simulink model "Control_planta_no_lineal_y_NN_mejor"  (R2023b)
settings: Solver=ode45  StartTime=0.0  StopTime=5000  RelTol=1e-3
values from neighbouring files (symbols this model uses):
  D = 0    [control_pid_tuning.m]
libraries: neural x98, simulink x9
(part 4 of 5)

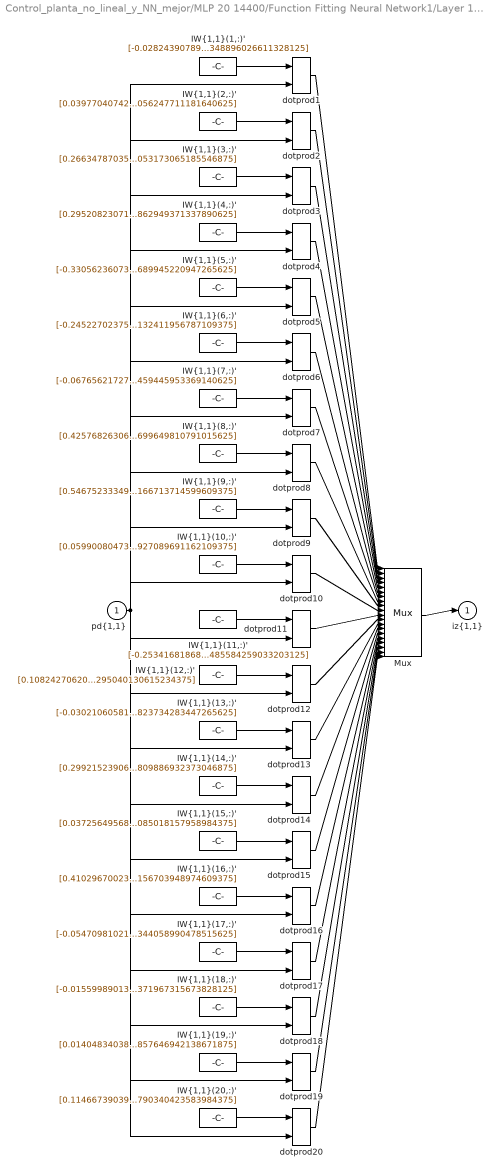
== system Control_planta_no_lineal_y_NN_mejor/MLP 20 14400/Function Fitting Neural Network1/Layer 1/IW{1,1} ==
  "pd{1,1}" : Inport  PortDimensions=11
      mask Display: e = 0.06;c1 = [120 230 180]/255;c2 = ([120 230 180]+0)/(256+128);c3 = ([120 230 180]+128)/(256+128);patch([0 1 1 0],[0 0 1 1],c1);patch([0 1 1 1-e 1-e 0+e],[0 0 1 1-e 0+e 0+e],c2);patch([0 0 1 1-e 0+e 0+e],[0 1 1 1-e 1-e 0+e],c3);plot([0 1 1 0 0],[0 0 1 1 0]);
  "IW{1,1}(1,:)'" : Constant  Value=[-0.028243907895395957419193422310854657553136348724365234375;0.005191973974844788126958849971970266778953373432159423828125;0.13337941289357180263408508835709653794765472412109375;0.069147078104058790071206885841093026101589202880859375;0.09470631313108242299581007728193071670830249786376953125;-0.0034271328340436456143247578864929892006330192089080810546875;0.04562563126758666098847783132441691122949123382568359375;-0.1381497395252362092588072073340299539268016815185546875;0.06431424914707263573721007787753478623926639556884765625;0.025641370199923095574146003627902246080338954925537109375;0.055434669391018993878095244554060627706348896026611328125]
      mask Display: e = 0.06;c1 = [120 150 230]/255;c2 = ([120 150 230]+0)/383;c3 = ([120 150 230]+128)/383;patch([0 1 1 0],[0 0 1 1],c1);patch([0 1 1 1-e 1-e 0+e],[0 0 1 1-e 0+e 0+e],c2);patch([0 0 1 1-e 0+e 0+e],[0 1 1 1-e 1-e 0+e],c3);plot([0 1 1 0 0],[0 0 1 1 0]);disp('Weights');
  "IW{1,1}(10,:)'" : Constant  Value=[0.059900804730095118244559415643379907123744487762451171875;0.0197715008122807678336840808697161264717578887939453125;0.04772829613961322714477120143783395178616046905517578125;-0.0932621366212354196978395748374168761074542999267578125;0.11487215483931519088844908083046902902424335479736328125;-0.0811079282463227635435742968184058554470539093017578125;-0.041933844459557438610897150965683977119624614715576171875;0.1459137174109600143534493099650717340409755706787109375;-0.0001450925426568216449439707727009363225079141557216644287109375;-0.007609474599997727468914110460218580556102097034454345703125;0.08578395140804272178680633942349231801927089691162109375]
      mask Display: e = 0.06;c1 = [120 150 230]/255;c2 = ([120 150 230]+0)/383;c3 = ([120 150 230]+128)/383;patch([0 1 1 0],[0 0 1 1],c1);patch([0 1 1 1-e 1-e 0+e],[0 0 1 1-e 0+e 0+e],c2);patch([0 0 1 1-e 0+e 0+e],[0 1 1 1-e 1-e 0+e],c3);plot([0 1 1 0 0],[0 0 1 1 0]);disp('Weights');
  "IW{1,1}(11,:)'" : Constant  Value=[-0.253416818681620303888024636762565933167934417724609375;0.052896434451703618073725721160371904261410236358642578125;0.068915348393704001228599054229562170803546905517578125;-0.09788049413072692772619376455622841604053974151611328125;0.057178838120491182195337387383915483951568603515625;0.10728410449795654224569574353154166601598262786865234375;0.0203502020408309301779947730892672552727162837982177734375;0.00125229069658645592207080188273948806454427540302276611328125;-0.14408483033475272261370037085725925862789154052734375;0.046135919620093245041569929298930219374597072601318359375;0.048354326720816971640903858542515081353485584259033203125]
      mask Display: e = 0.06;c1 = [120 150 230]/255;c2 = ([120 150 230]+0)/383;c3 = ([120 150 230]+128)/383;patch([0 1 1 0],[0 0 1 1],c1);patch([0 1 1 1-e 1-e 0+e],[0 0 1 1-e 0+e 0+e],c2);patch([0 0 1 1-e 0+e 0+e],[0 1 1 1-e 1-e 0+e],c3);plot([0 1 1 0 0],[0 0 1 1 0]);disp('Weights');
  "IW{1,1}(12,:)'" : Constant  Value=[0.1082427062098151038238569299210212193429470062255859375;-0.10783347592795040903457248759877984412014484405517578125;0.04932416990094290465407311785384081304073333740234375;0.1176909494571356240566473161379690282046794891357421875;0.056625605240315700361630746328955865465104579925537109375;0.125540484944335284378524875137372873723506927490234375;-0.009781079733660345831847138242665096186101436614990234375;0.0033784039907568054646180844002856247243471443653106689453125;-0.0201388726176935060896422413634354597888886928558349609375;-0.13223024952066808612727299987454898655414581298828125;0.106353782749821712538818019311293028295040130615234375]
      mask Display: e = 0.06;c1 = [120 150 230]/255;c2 = ([120 150 230]+0)/383;c3 = ([120 150 230]+128)/383;patch([0 1 1 0],[0 0 1 1],c1);patch([0 1 1 1-e 1-e 0+e],[0 0 1 1-e 0+e 0+e],c2);patch([0 0 1 1-e 0+e 0+e],[0 1 1 1-e 1-e 0+e],c3);plot([0 1 1 0 0],[0 0 1 1 0]);disp('Weights');
  "IW{1,1}(13,:)'" : Constant  Value=[-0.0302106058159601724433240832468072767369449138641357421875;-0.01083473636973667809935140127208796911872923374176025390625;0.00872722778809984812975475421126247965730726718902587890625;0.1694700438931255048746749025667668320238590240478515625;-0.055846650548267817715242244958062656223773956298828125;0.0683259083119855115118213007008307613432407379150390625;0.09901740039771596280093746145212207920849323272705078125;-0.0034830733886535903721937135202324498095549643039703369140625;0.086367876376208629896069624010124243795871734619140625;-0.0785352645771759394488498173814150504767894744873046875;0.11200836262547832211655673972927615977823734283447265625]
      mask Display: e = 0.06;c1 = [120 150 230]/255;c2 = ([120 150 230]+0)/383;c3 = ([120 150 230]+128)/383;patch([0 1 1 0],[0 0 1 1],c1);patch([0 1 1 1-e 1-e 0+e],[0 0 1 1-e 0+e 0+e],c2);patch([0 0 1 1-e 0+e 0+e],[0 1 1 1-e 1-e 0+e],c3);plot([0 1 1 0 0],[0 0 1 1 0]);disp('Weights');
  "IW{1,1}(14,:)'" : Constant  Value=[0.299215239064117122236297063864185474812984466552734375;-0.227303056462553942917992344519007019698619842529296875;-0.0246028750168633993100630874550915905274450778961181640625;0.0274141703222423004093766252253772108815610408782958984375;-0.0728212599418223138769690194749273359775543212890625;0.128567286087202525823869336818461306393146514892578125;-0.06510115768746389808274699362300452776253223419189453125;-0.0227893282940125098401384917679024511016905307769775390625;-0.0116248315098215031226924764951036195270717144012451171875;0.10342143834431290205788656066943076439201831817626953125;-0.057548270876921485406096934411834808997809886932373046875]
      mask Display: e = 0.06;c1 = [120 150 230]/255;c2 = ([120 150 230]+0)/383;c3 = ([120 150 230]+128)/383;patch([0 1 1 0],[0 0 1 1],c1);patch([0 1 1 1-e 1-e 0+e],[0 0 1 1-e 0+e 0+e],c2);patch([0 0 1 1-e 0+e 0+e],[0 1 1 1-e 1-e 0+e],c3);plot([0 1 1 0 0],[0 0 1 1 0]);disp('Weights');
  "IW{1,1}(15,:)'" : Constant  Value=[0.03725649568679145762217785886605270206928253173828125;0.058076084950603797107948622624462586827576160430908203125;-0.1269729602577863991630380269270972348749637603759765625;-0.01786746093381354205664734990932629443705081939697265625;-0.1569183017659522005882166695300838910043239593505859375;0.03235562642280716272313867420962196774780750274658203125;0.06457104482191818040082154084302601404488086700439453125;0.006190341039861292464496766996262522297911345958709716796875;-0.06269301714694208715883405602653510868549346923828125;-0.0645635039482781170061542752591776661574840545654296875;-0.103030060916822152616845187367289327085018157958984375]
      mask Display: e = 0.06;c1 = [120 150 230]/255;c2 = ([120 150 230]+0)/383;c3 = ([120 150 230]+128)/383;patch([0 1 1 0],[0 0 1 1],c1);patch([0 1 1 1-e 1-e 0+e],[0 0 1 1-e 0+e 0+e],c2);patch([0 0 1 1-e 0+e 0+e],[0 1 1 1-e 1-e 0+e],c3);plot([0 1 1 0 0],[0 0 1 1 0]);disp('Weights');
  "IW{1,1}(16,:)'" : Constant  Value=[0.41029670023388609134684656964964233338832855224609375;-0.054189782981134991535210332358474261127412319183349609375;-0.070172139747485762217849014632520265877246856689453125;-0.00901359172674678042758156237823641276918351650238037109375;-0.0008664644738628286997628169530116792884655296802520751953125;-0.0839314079297433790483040638719103299081325531005859375;-0.0105366135053931476994737437280491576530039310455322265625;0.0669426632220568584852316007527406327426433563232421875;-0.0782121647827017929532900097910896874964237213134765625;0.01064688551336578740957872213357404689304530620574951171875;0.0767344182627665849505405049058026634156703948974609375]
      mask Display: e = 0.06;c1 = [120 150 230]/255;c2 = ([120 150 230]+0)/383;c3 = ([120 150 230]+128)/383;patch([0 1 1 0],[0 0 1 1],c1);patch([0 1 1 1-e 1-e 0+e],[0 0 1 1-e 0+e 0+e],c2);patch([0 0 1 1-e 0+e 0+e],[0 1 1 1-e 1-e 0+e],c3);plot([0 1 1 0 0],[0 0 1 1 0]);disp('Weights');
  "IW{1,1}(17,:)'" : Constant  Value=[-0.054709810218583732055463997312472201883792877197265625;-0.058222078569764669497832443312290706671774387359619140625;0.0272915548239388953966066964085257495753467082977294921875;-0.002060889782607545385462177733870703377760946750640869140625;0.045200565384666151202974759826247463934123516082763671875;0.036566709240253382484642230565441423095762729644775390625;0.048434724470805601281853114414843730628490447998046875;0.1485881234961840269281907467302517034113407135009765625;-0.08280095269822450310126527028842247091233730316162109375;-0.01401815776626045596808811666278415941633284091949462890625;-0.100518799537367531371501172543503344058990478515625]
      mask Display: e = 0.06;c1 = [120 150 230]/255;c2 = ([120 150 230]+0)/383;c3 = ([120 150 230]+128)/383;patch([0 1 1 0],[0 0 1 1],c1);patch([0 1 1 1-e 1-e 0+e],[0 0 1 1-e 0+e 0+e],c2);patch([0 0 1 1-e 0+e 0+e],[0 1 1 1-e 1-e 0+e],c3);plot([0 1 1 0 0],[0 0 1 1 0]);disp('Weights');
  "IW{1,1}(18,:)'" : Constant  Value=[-0.01559989013582755400244561627687289728783071041107177734375;0.1058168090239341996294797354494221508502960205078125;-0.06821074930672578473522804642925621010363101959228515625;0.06328489319008401281507758540101349353790283203125;0.054756660574826011844695727859289036132395267486572265625;-0.053094792779526507608967023088553105480968952178955078125;0.025051428903148105498122077960942988283932209014892578125;-0.0230630997120841833847304513938070158474147319793701171875;0.159954775259797787878568442465621046721935272216796875;0.1668385232983627675107385357478051446378231048583984375;-0.1532613816918442228853791675646789371967315673828125]
      mask Display: e = 0.06;c1 = [120 150 230]/255;c2 = ([120 150 230]+0)/383;c3 = ([120 150 230]+128)/383;patch([0 1 1 0],[0 0 1 1],c1);patch([0 1 1 1-e 1-e 0+e],[0 0 1 1-e 0+e 0+e],c2);patch([0 0 1 1-e 0+e 0+e],[0 1 1 1-e 1-e 0+e],c3);plot([0 1 1 0 0],[0 0 1 1 0]);disp('Weights');
  "IW{1,1}(19,:)'" : Constant  Value=[0.01404834038980782608130315480821082019247114658355712890625;0.11681275441382070467977172256723861210048198699951171875;-0.074121670900885894273102394436136819422245025634765625;0.06853045999625316520020845700855716131627559661865234375;-0.0675103126368933048606635338728665374219417572021484375;0.10978393057352721362551761785653070546686649322509765625;-0.0695348327221847750667649279421311803162097930908203125;-0.07792378774692478027308339960654848255217075347900390625;0.03166961717159981481994890373243833892047405242919921875;0.10311534148308466873888988857288495637476444244384765625;-0.07671983312766754437017624468353460542857646942138671875]
      mask Display: e = 0.06;c1 = [120 150 230]/255;c2 = ([120 150 230]+0)/383;c3 = ([120 150 230]+128)/383;patch([0 1 1 0],[0 0 1 1],c1);patch([0 1 1 1-e 1-e 0+e],[0 0 1 1-e 0+e 0+e],c2);patch([0 0 1 1-e 0+e 0+e],[0 1 1 1-e 1-e 0+e],c3);plot([0 1 1 0 0],[0 0 1 1 0]);disp('Weights');
  "IW{1,1}(2,:)'" : Constant  Value=[0.039770407428281522033142181271614390425384044647216796875;-0.0245520760030410005458900712937975185923278331756591796875;0.03863350951806406030630824943727930076420307159423828125;0.117783072418614576104545221824082545936107635498046875;-0.091235315425064966721180326203466393053531646728515625;0.07428623396314408544593987926418776623904705047607421875;-0.076683739339302114945695620917831547558307647705078125;0.0269126755066263871618570391319735790602862834930419921875;-0.1583206985996788163095772006272454746067523956298828125;-0.166224771381416724924662275952869094908237457275390625;-0.0061015994473339052461824394413270056247711181640625]
      mask Display: e = 0.06;c1 = [120 150 230]/255;c2 = ([120 150 230]+0)/383;c3 = ([120 150 230]+128)/383;patch([0 1 1 0],[0 0 1 1],c1);patch([0 1 1 1-e 1-e 0+e],[0 0 1 1-e 0+e 0+e],c2);patch([0 0 1 1-e 0+e 0+e],[0 1 1 1-e 1-e 0+e],c3);plot([0 1 1 0 0],[0 0 1 1 0]);disp('Weights');
  "IW{1,1}(20,:)'" : Constant  Value=[0.11466739039623814744306429247444611974060535430908203125;-0.09303822905549240240841157856266363523900508880615234375;-0.0109706113092430633526586092330035171471536159515380859375;0.121986783925877972922791059318115003407001495361328125;0.005601834845350785012374483784469703095965087413787841796875;0.08696978354123073573500590782714425586163997650146484375;-0.0828842101220638449721178631079965271055698394775390625;-0.0932241771186295142825883885961957275867462158203125;0.049048714470215575012002062749161268584430217742919921875;0.0778398446714923253342277575939078815281391143798828125;0.0807200930695547158588709635296254418790340423583984375]
      mask Display: e = 0.06;c1 = [120 150 230]/255;c2 = ([120 150 230]+0)/383;c3 = ([120 150 230]+128)/383;patch([0 1 1 0],[0 0 1 1],c1);patch([0 1 1 1-e 1-e 0+e],[0 0 1 1-e 0+e 0+e],c2);patch([0 0 1 1-e 0+e 0+e],[0 1 1 1-e 1-e 0+e],c3);plot([0 1 1 0 0],[0 0 1 1 0]);disp('Weights');
  "IW{1,1}(3,:)'" : Constant  Value=[0.266347870359112837146398078402853570878505706787109375;-0.0671044057597638687884256114557501859962940216064453125;-0.060969763011602680358169692453884636051952838897705078125;0.010997470289914053342972266591459629125893115997314453125;0.053399938483572877145899582274068961851298809051513671875;-0.095813647433732052061117201446904800832271575927734375;-0.040191657564539844116335842727494309656322002410888671875;-0.007701322429141518356721096694172956631518900394439697265625;0.021981380257518508269942714150602114386856555938720703125;0.14104866807600335842920458162552677094936370849609375;-0.09012389593630169837279453304290655069053173065185546875]
      mask Display: e = 0.06;c1 = [120 150 230]/255;c2 = ([120 150 230]+0)/383;c3 = ([120 150 230]+128)/383;patch([0 1 1 0],[0 0 1 1],c1);patch([0 1 1 1-e 1-e 0+e],[0 0 1 1-e 0+e 0+e],c2);patch([0 0 1 1-e 0+e 0+e],[0 1 1 1-e 1-e 0+e],c3);plot([0 1 1 0 0],[0 0 1 1 0]);disp('Weights');
  "IW{1,1}(4,:)'" : Constant  Value=[0.2952082307138785832734129144228063523769378662109375;0.01231795472830080236115168901278593693859875202178955078125;0.02642149463240688056497873503758455626666545867919921875;0.03092587344321777453881594510676222853362560272216796875;-0.11677696579831486900502568460069596767425537109375;-0.11225588930709569368548983447908540256321430206298828125;-0.000808677190661592792432499354760011556209065020084381103515625;0.0276234412470428465635752246498668682761490345001220703125;-0.047124848593879144209584097779952571727335453033447265625;0.0734110199792780415695148121812962926924228668212890625;0.095929768161528594649922752068960107862949371337890625]
      mask Display: e = 0.06;c1 = [120 150 230]/255;c2 = ([120 150 230]+0)/383;c3 = ([120 150 230]+128)/383;patch([0 1 1 0],[0 0 1 1],c1);patch([0 1 1 1-e 1-e 0+e],[0 0 1 1-e 0+e 0+e],c2);patch([0 0 1 1-e 0+e 0+e],[0 1 1 1-e 1-e 0+e],c3);plot([0 1 1 0 0],[0 0 1 1 0]);disp('Weights');
  "IW{1,1}(5,:)'" : Constant  Value=[-0.33056236073119971141665018876665271818637847900390625;0.1875747485520468937902904826842132024466991424560546875;-0.024658968061582166308998154136133962310850620269775390625;0.01547521155301688315641950310919128241948783397674560546875;-0.0083768527854616130212672686639052699320018291473388671875;-0.0735477745604396215828302274530869908630847930908203125;-0.02162363177112518186628875582755426876246929168701171875;-0.04022877110090201935310716407911968417465686798095703125;0.1538088907838028041030753456652746535837650299072265625;0.017104904413551010045058120567773585207760334014892578125;0.06259815393081658019269752912805415689945220947265625]
      mask Display: e = 0.06;c1 = [120 150 230]/255;c2 = ([120 150 230]+0)/383;c3 = ([120 150 230]+128)/383;patch([0 1 1 0],[0 0 1 1],c1);patch([0 1 1 1-e 1-e 0+e],[0 0 1 1-e 0+e 0+e],c2);patch([0 0 1 1-e 0+e 0+e],[0 1 1 1-e 1-e 0+e],c3);plot([0 1 1 0 0],[0 0 1 1 0]);disp('Weights');
  "IW{1,1}(6,:)'" : Constant  Value=[-0.24522702375562810406250946471118368208408355712890625;-0.0308170360453197123007385016535408794879913330078125;-0.1152032330723841424546805001227767206728458404541015625;0.1210684922289272102968737954142852686345577239990234375;0.0099718051373125400627106529327647876925766468048095703125;-0.055898296203996007680547819518324104137718677520751953125;-0.06781583096636688290370642562265857122838497161865234375;0.1345922742042022501873788087323191575706005096435546875;0.0297068174305298686455056866861923481337726116180419921875;0.025479370583105502567899947052865172736346721649169921875;0.0871667663205045462060382988056517206132411956787109375]
      mask Display: e = 0.06;c1 = [120 150 230]/255;c2 = ([120 150 230]+0)/383;c3 = ([120 150 230]+128)/383;patch([0 1 1 0],[0 0 1 1],c1);patch([0 1 1 1-e 1-e 0+e],[0 0 1 1-e 0+e 0+e],c2);patch([0 0 1 1-e 0+e 0+e],[0 1 1 1-e 1-e 0+e],c3);plot([0 1 1 0 0],[0 0 1 1 0]);disp('Weights');
  "IW{1,1}(7,:)'" : Constant  Value=[-0.06765621727002278651408317955429083667695522308349609375;-0.0553547130583876001441723246898618526756763458251953125;-0.0802669371512219897990547679000883363187313079833984375;0.1425949581192766102422098128954530693590641021728515625;0.008009784174367172437936091000665328465402126312255859375;0.044256063428620144584169082691005314700305461883544921875;0.021906829266177839377061076220343238674104213714599609375;0.0296145069756109900749319052692953846417367458343505859375;-0.01513404668814787197572702126535659772343933582305908203125;0.1655381443596699586606746379402466118335723876953125;0.10528093902201775267091221621740260161459445953369140625]
      mask Display: e = 0.06;c1 = [120 150 230]/255;c2 = ([120 150 230]+0)/383;c3 = ([120 150 230]+128)/383;patch([0 1 1 0],[0 0 1 1],c1);patch([0 1 1 1-e 1-e 0+e],[0 0 1 1-e 0+e 0+e],c2);patch([0 0 1 1-e 0+e 0+e],[0 1 1 1-e 1-e 0+e],c3);plot([0 1 1 0 0],[0 0 1 1 0]);disp('Weights');
  "IW{1,1}(8,:)'" : Constant  Value=[0.425768263063369400978075418606749735772609710693359375;-0.2993624824245733062610952401882968842983245849609375;-0.038008311061219178517145422802059329114854335784912109375;-0.000703385241561246972973042712595770353800617158412933349609375;0.0991174010007415950962439410432125441730022430419921875;-0.0765070769917539639237702431273646652698516845703125;0.03518023643958355373140278743449016474187374114990234375;0.0099877833459521177250639567546386388130486011505126953125;0.087648756451609965978377658757381141185760498046875;-0.0830457746408952146577320263531873933970928192138671875;-0.0710771829620092943091691495283157564699649810791015625]
      mask Display: e = 0.06;c1 = [120 150 230]/255;c2 = ([120 150 230]+0)/383;c3 = ([120 150 230]+128)/383;patch([0 1 1 0],[0 0 1 1],c1);patch([0 1 1 1-e 1-e 0+e],[0 0 1 1-e 0+e 0+e],c2);patch([0 0 1 1-e 0+e 0+e],[0 1 1 1-e 1-e 0+e],c3);plot([0 1 1 0 0],[0 0 1 1 0]);disp('Weights');
  "IW{1,1}(9,:)'" : Constant  Value=[0.54675233349644181135573717256193049252033233642578125;-0.412741138687774233861915718080126680433750152587890625;-0.10487264071427380984768973348764120601117610931396484375;0.138693990933245359098435756095568649470806121826171875;-0.005549763080092340837567999045631950139068067073822021484375;-0.00697363471678230130434972267039483995176851749420166015625;0.0677740304076877853045601796111441217362880706787109375;-0.059259882919453159277889398026673006825149059295654296875;0.042463366677406189086951826539007015526294708251953125;-0.060735496643573971820018186917877756059169769287109375;0.0661040701535159092028237637350684963166713714599609375]
      mask Display: e = 0.06;c1 = [120 150 230]/255;c2 = ([120 150 230]+0)/383;c3 = ([120 150 230]+128)/383;patch([0 1 1 0],[0 0 1 1],c1);patch([0 1 1 1-e 1-e 0+e],[0 0 1 1-e 0+e 0+e],c2);patch([0 0 1 1-e 0+e 0+e],[0 1 1 1-e 1-e 0+e],c3);plot([0 1 1 0 0],[0 0 1 1 0]);disp('Weights');
  Mux : Mux  Inputs=20
      mask Display: e = 0.06;c1 = [120 150 230]/255;c2 = ([120 150 230]+0)/383;c3 = ([120 150 230]+128)/383;patch([0 1 1 0],[0 0 1 1],c1);patch([0 1 1 1-e 1-e 0+e],[0 0 1 1-e 0+e 0+e],c2);patch([0 0 1 1-e 0+e 0+e],[0 1 1 1-e 1-e 0+e],c3);plot([0 1 1 0 0],[0 0 1 1 0]);disp('Mux');
  dotprod{1..20} (20 alike) : neural/Weight Functions/dotprod
  "iz{1,1}" : Outport
      mask Display: e = 0.06;c1 = [120 230 180]/255;c2 = ([120 230 180]+0)/(256+128);c3 = ([120 230 180]+128)/(256+128);patch([0 1 1 0],[0 0 1 1],c1);patch([0 1 1 1-e 1-e 0+e],[0 0 1 1-e 0+e 0+e],c2);patch([0 0 1 1-e 0+e 0+e],[0 1 1 1-e 1-e 0+e],c3);plot([0 1 1 0 0],[0 0 1 1 0]);
  wires:
  "IW{1,1}(1,:)'"/1 -> dotprod1/1
  "pd{1,1}"/1 -> dotprod1/2, dotprod2/2, dotprod3/2, dotprod4/2, dotprod5/2, dotprod6/2, dotprod7/2, dotprod8/2, dotprod9/2, dotprod10/2, dotprod11/2, dotprod12/2, dotprod13/2, dotprod14/2, dotprod15/2, dotprod16/2, dotprod17/2, dotprod18/2, dotprod19/2, dotprod20/2
  dotprod1/1 -> Mux/1
  "IW{1,1}(2,:)'"/1 -> dotprod2/1
  dotprod2/1 -> Mux/2
  "IW{1,1}(3,:)'"/1 -> dotprod3/1
  dotprod3/1 -> Mux/3
  "IW{1,1}(4,:)'"/1 -> dotprod4/1
  dotprod4/1 -> Mux/4
  "IW{1,1}(5,:)'"/1 -> dotprod5/1
  dotprod5/1 -> Mux/5
  "IW{1,1}(6,:)'"/1 -> dotprod6/1
  dotprod6/1 -> Mux/6
  "IW{1,1}(7,:)'"/1 -> dotprod7/1
  dotprod7/1 -> Mux/7
  "IW{1,1}(8,:)'"/1 -> dotprod8/1
  dotprod8/1 -> Mux/8
  "IW{1,1}(9,:)'"/1 -> dotprod9/1
  dotprod9/1 -> Mux/9
  "IW{1,1}(10,:)'"/1 -> dotprod10/1
  dotprod10/1 -> Mux/10
  "IW{1,1}(11,:)'"/1 -> dotprod11/1
  dotprod11/1 -> Mux/11
  "IW{1,1}(12,:)'"/1 -> dotprod12/1
  dotprod12/1 -> Mux/12
  "IW{1,1}(13,:)'"/1 -> dotprod13/1
  dotprod13/1 -> Mux/13
  "IW{1,1}(14,:)'"/1 -> dotprod14/1
  dotprod14/1 -> Mux/14
  "IW{1,1}(15,:)'"/1 -> dotprod15/1
  dotprod15/1 -> Mux/15
  "IW{1,1}(16,:)'"/1 -> dotprod16/1
  dotprod16/1 -> Mux/16
  "IW{1,1}(17,:)'"/1 -> dotprod17/1
  dotprod17/1 -> Mux/17
  "IW{1,1}(18,:)'"/1 -> dotprod18/1
  dotprod18/1 -> Mux/18
  "IW{1,1}(19,:)'"/1 -> dotprod19/1
  dotprod19/1 -> Mux/19
  "IW{1,1}(20,:)'"/1 -> dotprod20/1
  dotprod20/1 -> Mux/20
  Mux/1 -> "iz{1,1}"/1

== system Control_planta_no_lineal_y_NN_mejor/MLP 20 14400/Function Fitting Neural Network1/Layer 2/Delays 1 ==
  "p{2}" : Inport  PortDimensions=20
      mask Display: e = 0.06;c1 = [120 230 180]/255;c2 = ([120 230 180]+0)/(256+128);c3 = ([120 230 180]+128)/(256+128);patch([0 1 1 0],[0 0 1 1],c1);patch([0 1 1 1-e 1-e 0+e],[0 0 1 1-e 0+e 0+e],c2);patch([0 0 1 1-e 0+e 0+e],[0 1 1 1-e 1-e 0+e],c3);plot([0 1 1 0 0],[0 0 1 1 0]);
  mux : Mux  Inputs=1
      mask Display: e = 0.06;c1 = [120 150 230]/255;c2 = ([120 150 230]+0)/383;c3 = ([120 150 230]+128)/383;patch([0 1 1 0],[0 0 1 1],c1);patch([0 1 1 1-e 1-e 0+e],[0 0 1 1-e 0+e 0+e],c2);patch([0 0 1 1-e 0+e 0+e],[0 1 1 1-e 1-e 0+e],c3);plot([0 1 1 0 0],[0 0 1 1 0]);disp('Mux')
  "pd{2,1}" : Outport
      mask Display: e = 0.06;c1 = [120 230 180]/255;c2 = ([120 230 180]+0)/(256+128);c3 = ([120 230 180]+128)/(256+128);patch([0 1 1 0],[0 0 1 1],c1);patch([0 1 1 1-e 1-e 0+e],[0 0 1 1-e 0+e 0+e],c2);patch([0 0 1 1-e 0+e 0+e],[0 1 1 1-e 1-e 0+e],c3);plot([0 1 1 0 0],[0 0 1 1 0]);
  wires:
  "p{2}"/1 -> mux/1
  mux/1 -> "pd{2,1}"/1

== system Control_planta_no_lineal_y_NN_mejor/MLP 20 14400/Function Fitting Neural Network1/Layer 2/LW{2,1} ==
  "ad{2,1}" : Inport  PortDimensions=20
      mask Display: e = 0.06;c1 = [120 230 180]/255;c2 = ([120 230 180]+0)/(256+128);c3 = ([120 230 180]+128)/(256+128);patch([0 1 1 0],[0 0 1 1],c1);patch([0 1 1 1-e 1-e 0+e],[0 0 1 1-e 0+e 0+e],c2);patch([0 0 1 1-e 0+e 0+e],[0 1 1 1-e 1-e 0+e],c3);plot([0 1 1 0 0],[0 0 1 1 0]);
  "IW{2,1}(1,:)'" : Constant  Value=[1.0308324817309266752118901422363705933094024658203125;-0.42793371893883047629714155846158973872661590576171875;0.9857391162526456529491269975551404058933258056640625;0.65288972697485758711621883776388131082057952880859375;-1.0698277001364495664148535070125944912433624267578125;-1.0731197870900153201745297337765805423259735107421875;0.50410824546317822836272171116434037685394287109375;1.061189879303181538006128903361968696117401123046875;1.4729402418759407478177081429748795926570892333984375;-0.1759553217513047940201431629247963428497314453125;-0.84066043357673703173560397772234864532947540283203125;0.66490271328374273007710826277616433799266815185546875;0.773816549352292160079969107755459845066070556640625;0.6930009350234882514740775150130502879619598388671875;-0.8395888854185000749197342884144745767116546630859375;1.2423075825811722427971517390687949955463409423828125;0.8668323116487035573385355746722780168056488037109375;-0.06581321559824666878046883766728569753468036651611328125;1.3136860251400792609643985997536219656467437744140625;0.69992464043873814372176411779946647584438323974609375]
      mask Display: e = 0.06;c1 = [120 150 230]/255;c2 = ([120 150 230]+0)/383;c3 = ([120 150 230]+128)/383;patch([0 1 1 0],[0 0 1 1],c1);patch([0 1 1 1-e 1-e 0+e],[0 0 1 1-e 0+e 0+e],c2);patch([0 0 1 1-e 0+e 0+e],[0 1 1 1-e 1-e 0+e],c3);plot([0 1 1 0 0],[0 0 1 1 0]);disp('weights');
  Mux : Mux  Inputs=1
      mask Display: e = 0.06;c1 = [120 150 230]/255;c2 = ([120 150 230]+0)/383;c3 = ([120 150 230]+128)/383;patch([0 1 1 0],[0 0 1 1],c1);patch([0 1 1 1-e 1-e 0+e],[0 0 1 1-e 0+e 0+e],c2);patch([0 0 1 1-e 0+e 0+e],[0 1 1 1-e 1-e 0+e],c3);plot([0 1 1 0 0],[0 0 1 1 0]);disp('Mux');
  dotprod1 : neural/Weight Functions/dotprod
  "lz{2,1}" : Outport
      mask Display: e = 0.06;c1 = [120 230 180]/255;c2 = ([120 230 180]+0)/(256+128);c3 = ([120 230 180]+128)/(256+128);patch([0 1 1 0],[0 0 1 1],c1);patch([0 1 1 1-e 1-e 0+e],[0 0 1 1-e 0+e 0+e],c2);patch([0 0 1 1-e 0+e 0+e],[0 1 1 1-e 1-e 0+e],c3);plot([0 1 1 0 0],[0 0 1 1 0]);
  wires:
  "IW{2,1}(1,:)'"/1 -> dotprod1/1
  "ad{2,1}"/1 -> dotprod1/2
  dotprod1/1 -> Mux/1
  Mux/1 -> "lz{2,1}"/1

== system Control_planta_no_lineal_y_NN_mejor/MLP 20 3600/Function Fitting Neural Network/Layer 1/Delays 1 ==
  "p{1}" : Inport  PortDimensions=11
      mask Display: e = 0.06;c1 = [120 230 180]/255;c2 = ([120 230 180]+0)/(256+128);c3 = ([120 230 180]+128)/(256+128);patch([0 1 1 0],[0 0 1 1],c1);patch([0 1 1 1-e 1-e 0+e],[0 0 1 1-e 0+e 0+e],c2);patch([0 0 1 1-e 0+e 0+e],[0 1 1 1-e 1-e 0+e],c3);plot([0 1 1 0 0],[0 0 1 1 0]);
  mux : Mux  Inputs=1
      mask Display: e = 0.06;c1 = [120 150 230]/255;c2 = ([120 150 230]+0)/383;c3 = ([120 150 230]+128)/383;patch([0 1 1 0],[0 0 1 1],c1);patch([0 1 1 1-e 1-e 0+e],[0 0 1 1-e 0+e 0+e],c2);patch([0 0 1 1-e 0+e 0+e],[0 1 1 1-e 1-e 0+e],c3);plot([0 1 1 0 0],[0 0 1 1 0]);disp('Mux')
  "pd{1,1}" : Outport
      mask Display: e = 0.06;c1 = [120 230 180]/255;c2 = ([120 230 180]+0)/(256+128);c3 = ([120 230 180]+128)/(256+128);patch([0 1 1 0],[0 0 1 1],c1);patch([0 1 1 1-e 1-e 0+e],[0 0 1 1-e 0+e 0+e],c2);patch([0 0 1 1-e 0+e 0+e],[0 1 1 1-e 1-e 0+e],c3);plot([0 1 1 0 0],[0 0 1 1 0]);
  wires:
  "p{1}"/1 -> mux/1
  mux/1 -> "pd{1,1}"/1

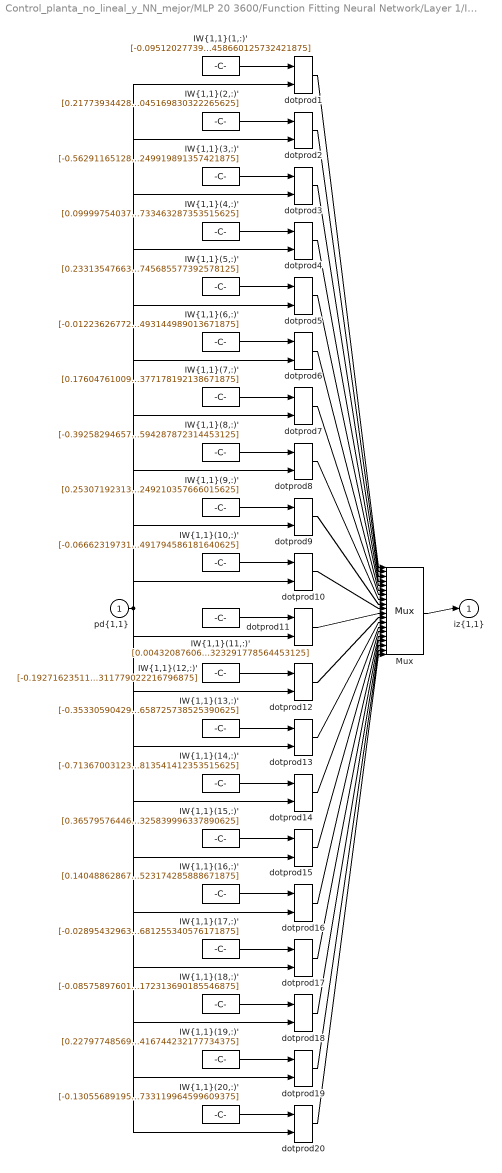
== system Control_planta_no_lineal_y_NN_mejor/MLP 20 3600/Function Fitting Neural Network/Layer 1/IW{1,1} ==
  "pd{1,1}" : Inport  PortDimensions=11
      mask Display: e = 0.06;c1 = [120 230 180]/255;c2 = ([120 230 180]+0)/(256+128);c3 = ([120 230 180]+128)/(256+128);patch([0 1 1 0],[0 0 1 1],c1);patch([0 1 1 1-e 1-e 0+e],[0 0 1 1-e 0+e 0+e],c2);patch([0 0 1 1-e 0+e 0+e],[0 1 1 1-e 1-e 0+e],c3);plot([0 1 1 0 0],[0 0 1 1 0]);
  "IW{1,1}(1,:)'" : Constant  Value=[-0.09512027739777671742071873950408189557492733001708984375;0.2204798602969697263187498492698068730533123016357421875;0.1693389750250708647438813159169512800872325897216796875;0.15999744215939204483589719529845751821994781494140625;-0.0130764518279639953279858133328161784447729587554931640625;0.24744973904865741332059769774787127971649169921875;0.032477541497795192615427595228538848459720611572265625;-0.112158380930051093660182459643692709505558013916015625;-0.2060854519390003247725218216146458871662616729736328125;-0.07677540605744311019709158472323906607925891876220703125;-0.28261245258007583469606061044032685458660125732421875]
      mask Display: e = 0.06;c1 = [120 150 230]/255;c2 = ([120 150 230]+0)/383;c3 = ([120 150 230]+128)/383;patch([0 1 1 0],[0 0 1 1],c1);patch([0 1 1 1-e 1-e 0+e],[0 0 1 1-e 0+e 0+e],c2);patch([0 0 1 1-e 0+e 0+e],[0 1 1 1-e 1-e 0+e],c3);plot([0 1 1 0 0],[0 0 1 1 0]);disp('Weights');
  "IW{1,1}(10,:)'" : Constant  Value=[-0.0666231973122941301124200208505499176681041717529296875;-0.2017198475688135872463391251585562713444232940673828125;-0.131403352519076921378626821024226956069469451904296875;0.0680218762872189242063569736274075694382190704345703125;-0.121483209919828250011875070413225330412387847900390625;-0.10799945881927419666368450634763576090335845947265625;0.042464037699283453675125343806939781643450260162353515625;0.13660098615683036182844034556183032691478729248046875;-0.048813771901668238928362342221589642576873302459716796875;-0.001603538647608613275374889184377025230787694454193115234375;0.136278237911712951646592273391433991491794586181640625]
      mask Display: e = 0.06;c1 = [120 150 230]/255;c2 = ([120 150 230]+0)/383;c3 = ([120 150 230]+128)/383;patch([0 1 1 0],[0 0 1 1],c1);patch([0 1 1 1-e 1-e 0+e],[0 0 1 1-e 0+e 0+e],c2);patch([0 0 1 1-e 0+e 0+e],[0 1 1 1-e 1-e 0+e],c3);plot([0 1 1 0 0],[0 0 1 1 0]);disp('Weights');
  "IW{1,1}(11,:)'" : Constant  Value=[0.00432087606357412119806316042058824677951633930206298828125;-0.0176952600575759240453255216607431066222488880157470703125;-0.213305144502392185490435849715140648186206817626953125;-0.0070486602151344224242990321727120317518711090087890625;-0.05364586495172600499881099267440731637179851531982421875;0.07767434866176943508708774288606946356594562530517578125;-0.0971338379072229918254066660665557719767093658447265625;0.207955773723864589808130176606937311589717864990234375;0.1294664906229296974515818874351680278778076171875;0.2660154298495494007426032112562097609043121337890625;-0.073358618432946276488593184694764204323291778564453125]
      mask Display: e = 0.06;c1 = [120 150 230]/255;c2 = ([120 150 230]+0)/383;c3 = ([120 150 230]+128)/383;patch([0 1 1 0],[0 0 1 1],c1);patch([0 1 1 1-e 1-e 0+e],[0 0 1 1-e 0+e 0+e],c2);patch([0 0 1 1-e 0+e 0+e],[0 1 1 1-e 1-e 0+e],c3);plot([0 1 1 0 0],[0 0 1 1 0]);disp('Weights');
  "IW{1,1}(12,:)'" : Constant  Value=[-0.19271623511614344170794765886967070400714874267578125;-0.0184345089596978893575762725731692626141011714935302734375;0.1818671103665819577255291505935019813477993011474609375;0.17976642257001118618831014828174374997615814208984375;-0.32683263902470838235814198924344964325428009033203125;0.0300403416657621137597633520499584847129881381988525390625;-0.216759225621790452276371752304839901626110076904296875;0.09582118151532288685690019747198675759136676788330078125;-0.09946574593348835036099586659474880434572696685791015625;0.07014872665288897357616093586329952813684940338134765625;0.02873562751153151129113183515073615126311779022216796875]
      mask Display: e = 0.06;c1 = [120 150 230]/255;c2 = ([120 150 230]+0)/383;c3 = ([120 150 230]+128)/383;patch([0 1 1 0],[0 0 1 1],c1);patch([0 1 1 1-e 1-e 0+e],[0 0 1 1-e 0+e 0+e],c2);patch([0 0 1 1-e 0+e 0+e],[0 1 1 1-e 1-e 0+e],c3);plot([0 1 1 0 0],[0 0 1 1 0]);disp('Weights');
  "IW{1,1}(13,:)'" : Constant  Value=[-0.353305904295088402111701952890143729746341705322265625;0.1972997021875265433177304430500953458249568939208984375;-0.2012460995410638997515917480995994992554187774658203125;0.0301829712379165400470970581636720453388988971710205078125;0.2089684975410117939720322510765981860458850860595703125;0.044235490321654170886578327781535335816442966461181640625;0.0017528284320446735865262066766945281415246427059173583984375;-0.10454125614091246132542067925896844826638698577880859375;0.13757552464859423846377239897265098989009857177734375;0.218120715272192400302486703367321752011775970458984375;-0.0680255667008539399720490337131195701658725738525390625]
      mask Display: e = 0.06;c1 = [120 150 230]/255;c2 = ([120 150 230]+0)/383;c3 = ([120 150 230]+128)/383;patch([0 1 1 0],[0 0 1 1],c1);patch([0 1 1 1-e 1-e 0+e],[0 0 1 1-e 0+e 0+e],c2);patch([0 0 1 1-e 0+e 0+e],[0 1 1 1-e 1-e 0+e],c3);plot([0 1 1 0 0],[0 0 1 1 0]);disp('Weights');
  "IW{1,1}(14,:)'" : Constant  Value=[-0.71367003123356032023849593315389938652515411376953125;0.50319007364462631226587063792976550757884979248046875;0.1722942567524924084576554150771698914468288421630859375;0.08568542920109976923637162826707935892045497894287109375;-0.37503742238744719461607246557832695543766021728515625;0.1768643526710487468012189538058009929955005645751953125;0.0232124438195507043491971899129566736519336700439453125;0.003472048340225260439073640128526676562614738941192626953125;0.06760192997916190937868208266081637702882289886474609375;-0.08959089375883240446984956406595301814377307891845703125;-0.06922431239184691220689416013556183315813541412353515625]
      mask Display: e = 0.06;c1 = [120 150 230]/255;c2 = ([120 150 230]+0)/383;c3 = ([120 150 230]+128)/383;patch([0 1 1 0],[0 0 1 1],c1);patch([0 1 1 1-e 1-e 0+e],[0 0 1 1-e 0+e 0+e],c2);patch([0 0 1 1-e 0+e 0+e],[0 1 1 1-e 1-e 0+e],c3);plot([0 1 1 0 0],[0 0 1 1 0]);disp('Weights');
  "IW{1,1}(15,:)'" : Constant  Value=[0.365795764462425954111068904239800758659839630126953125;0.06729310570741513231052266519327531568706035614013671875;-0.2147062380224042943410722728003747761249542236328125;0.048742591759215726787690670107622281648218631744384765625;-0.10890129208302791463669478844167315401136875152587890625;0.0898214300034483326129475244670175015926361083984375;-0.15083645725684602378890986074111424386501312255859375;-0.14781908076151217823479555590893141925334930419921875;0.2702565728639771958086157610523514449596405029296875;0.06007461867822545820150281770111178047955036163330078125;0.039742536380477179458470260442481958307325839996337890625]
      mask Display: e = 0.06;c1 = [120 150 230]/255;c2 = ([120 150 230]+0)/383;c3 = ([120 150 230]+128)/383;patch([0 1 1 0],[0 0 1 1],c1);patch([0 1 1 1-e 1-e 0+e],[0 0 1 1-e 0+e 0+e],c2);patch([0 0 1 1-e 0+e 0+e],[0 1 1 1-e 1-e 0+e],c3);plot([0 1 1 0 0],[0 0 1 1 0]);disp('Weights');
  "IW{1,1}(16,:)'" : Constant  Value=[0.1404886286757351110399127946948283351957798004150390625;0.248162714513551818651393432446639053523540496826171875;0.31757755194244896568278591075795702636241912841796875;-0.00511038491646554661473889069611686863936483860015869140625;-0.04387131909707374377571653667473583482205867767333984375;-0.1738187968821733875302015803754329681396484375;0.070420272003217043721434720282559283077716827392578125;-0.0240012295763493178901715197071098373271524906158447265625;0.048100153168631358535645148322146269492805004119873046875;-0.08195867578675473941185458670588559471070766448974609375;-0.330876539492720223023525250027887523174285888671875]
      mask Display: e = 0.06;c1 = [120 150 230]/255;c2 = ([120 150 230]+0)/383;c3 = ([120 150 230]+128)/383;patch([0 1 1 0],[0 0 1 1],c1);patch([0 1 1 1-e 1-e 0+e],[0 0 1 1-e 0+e 0+e],c2);patch([0 0 1 1-e 0+e 0+e],[0 1 1 1-e 1-e 0+e],c3);plot([0 1 1 0 0],[0 0 1 1 0]);disp('Weights');
  "IW{1,1}(17,:)'" : Constant  Value=[-0.028954329638684495051847989088855683803558349609375;-0.0721551449907472941536212829305441118776798248291015625;0.1610778363038999072553991709355614148080348968505859375;0.231394913003747426660794417330180294811725616455078125;-0.145183632266966344825931400919216684997081756591796875;-0.1886653245576965509666678144640172831714153289794921875;-0.130403753831254187733890148592763580381870269775390625;-0.07640396967507358250148996603456907905638217926025390625;-0.06337778154152444443081293456998537294566631317138671875;0.1359718729747601273505352992287953384220600128173828125;0.3668193456582755640482673697988502681255340576171875]
      mask Display: e = 0.06;c1 = [120 150 230]/255;c2 = ([120 150 230]+0)/383;c3 = ([120 150 230]+128)/383;patch([0 1 1 0],[0 0 1 1],c1);patch([0 1 1 1-e 1-e 0+e],[0 0 1 1-e 0+e 0+e],c2);patch([0 0 1 1-e 0+e 0+e],[0 1 1 1-e 1-e 0+e],c3);plot([0 1 1 0 0],[0 0 1 1 0]);disp('Weights');
  "IW{1,1}(18,:)'" : Constant  Value=[-0.08575897601754457755252047945759841240942478179931640625;0.10453601950626341399175345259209279902279376983642578125;-0.007335713426279331927926108392057358287274837493896484375;-0.2381456579383970650898305621012696065008640289306640625;-0.0143591331657741440308573288575644255615770816802978515625;0.262629005134863480197537910498795099556446075439453125;-0.067902562981049296997326791824889369308948516845703125;-0.186700327777929497852227314069750718772411346435546875;-0.2160664927715998662183238820944097824394702911376953125;0.09512254646240762834263904323961469344794750213623046875;-0.00987881573437514315383367602407815866172313690185546875]
      mask Display: e = 0.06;c1 = [120 150 230]/255;c2 = ([120 150 230]+0)/383;c3 = ([120 150 230]+128)/383;patch([0 1 1 0],[0 0 1 1],c1);patch([0 1 1 1-e 1-e 0+e],[0 0 1 1-e 0+e 0+e],c2);patch([0 0 1 1-e 0+e 0+e],[0 1 1 1-e 1-e 0+e],c3);plot([0 1 1 0 0],[0 0 1 1 0]);disp('Weights');
  "IW{1,1}(19,:)'" : Constant  Value=[0.2279774856972925090037307427337509579956531524658203125;-0.1528454839187013691859107211712398566305637359619140625;-0.0296888052415651935989071574795161723159253597259521484375;-0.1897884112687858448875743988537578843533992767333984375;-0.09657158632854666302502977259791805408895015716552734375;-0.1753218722240685589763842244792613200843334197998046875;0.010106046362199617993926636927426443435251712799072265625;-0.17249125111803687016021058298065327107906341552734375;0.0182418690404831072837676941844620159827172756195068359375;-0.2191919341265579912469974033228936605155467987060546875;-0.4071472354185112774160870685591362416744232177734375]
      mask Display: e = 0.06;c1 = [120 150 230]/255;c2 = ([120 150 230]+0)/383;c3 = ([120 150 230]+128)/383;patch([0 1 1 0],[0 0 1 1],c1);patch([0 1 1 1-e 1-e 0+e],[0 0 1 1-e 0+e 0+e],c2);patch([0 0 1 1-e 0+e 0+e],[0 1 1 1-e 1-e 0+e],c3);plot([0 1 1 0 0],[0 0 1 1 0]);disp('Weights');
  "IW{1,1}(2,:)'" : Constant  Value=[0.217739344280909741247143074360792525112628936767578125;0.1729156536563728197020139987216680310666561126708984375;-0.01314001404934124483947499584246543236076831817626953125;-0.1970889302021514577489824660005979239940643310546875;0.1657430732697456055024787247020867653191089630126953125;-0.19565476628002020920149561789003200829029083251953125;0.17828638803165552939589133529807440936565399169921875;0.06779651317808876864745570856030099093914031982421875;0.059611287458772581338006801843221182934939861297607421875;-0.1782270532617640512729195734209497459232807159423828125;0.07741134691830343916851830954328761436045169830322265625]
      mask Display: e = 0.06;c1 = [120 150 230]/255;c2 = ([120 150 230]+0)/383;c3 = ([120 150 230]+128)/383;patch([0 1 1 0],[0 0 1 1],c1);patch([0 1 1 1-e 1-e 0+e],[0 0 1 1-e 0+e 0+e],c2);patch([0 0 1 1-e 0+e 0+e],[0 1 1 1-e 1-e 0+e],c3);plot([0 1 1 0 0],[0 0 1 1 0]);disp('Weights');
  "IW{1,1}(20,:)'" : Constant  Value=[-0.13055689195591380080685439679655246436595916748046875;-0.131556933987213409142924547268194146454334259033203125;-0.117056744366267562185157657950185239315032958984375;-0.067986220932443275355439027407555840909481048583984375;0.248074701417002441150572167316568084061145782470703125;-0.118037412195859225949590154414181597530841827392578125;-0.0270311783106162127621185931047875783406198024749755859375;0.044076136896465424597213456081590265966951847076416015625;0.18559473931613801322981771591003052890300750732421875;-0.009449873611358385050440489294487633742392063140869140625;-0.257528338746100649014891814658767543733119964599609375]
      mask Display: e = 0.06;c1 = [120 150 230]/255;c2 = ([120 150 230]+0)/383;c3 = ([120 150 230]+128)/383;patch([0 1 1 0],[0 0 1 1],c1);patch([0 1 1 1-e 1-e 0+e],[0 0 1 1-e 0+e 0+e],c2);patch([0 0 1 1-e 0+e 0+e],[0 1 1 1-e 1-e 0+e],c3);plot([0 1 1 0 0],[0 0 1 1 0]);disp('Weights');
  "IW{1,1}(3,:)'" : Constant  Value=[-0.56291165128348852331185980801819823682308197021484375;0.25648678641237332431757067752187140285968780517578125;0.055225659156198196597653549133610795252025127410888671875;-0.26847948487825290531105792979360558092594146728515625;0.10200280465687792952333978746537468396127223968505859375;0.09790783300398896160654516052090912126004695892333984375;0.059793268603445699771459231897097197361290454864501953125;-0.1501034713150407318149603952406323514878749847412109375;0.0110726462146306971201514812719324254430830478668212890625;0.07248031451935228741678685082661104388535022735595703125;0.08162174380879543000855136369864339940249919891357421875]
      mask Display: e = 0.06;c1 = [120 150 230]/255;c2 = ([120 150 230]+0)/383;c3 = ([120 150 230]+128)/383;patch([0 1 1 0],[0 0 1 1],c1);patch([0 1 1 1-e 1-e 0+e],[0 0 1 1-e 0+e 0+e],c2);patch([0 0 1 1-e 0+e 0+e],[0 1 1 1-e 1-e 0+e],c3);plot([0 1 1 0 0],[0 0 1 1 0]);disp('Weights');
  "IW{1,1}(4,:)'" : Constant  Value=[0.0999975403705496701523003366673947311937808990478515625;-0.24043794877549473643085775620420463383197784423828125;0.1447891991252030774450787475871038623154163360595703125;-0.02898362210312743769691223860718309879302978515625;-0.2259766990698166555517900633276440203189849853515625;-0.112874866778603200057062849737121723592281341552734375;-0.1367826068889311519338747302754200063645839691162109375;0.1493051679981612644976252113337977789342403411865234375;0.09252979115524019582128545380328432656824588775634765625;-0.1350909714089480739840354317493620328605175018310546875;-0.1577116928526821892919684842127026058733463287353515625]
      mask Display: e = 0.06;c1 = [120 150 230]/255;c2 = ([120 150 230]+0)/383;c3 = ([120 150 230]+128)/383;patch([0 1 1 0],[0 0 1 1],c1);patch([0 1 1 1-e 1-e 0+e],[0 0 1 1-e 0+e 0+e],c2);patch([0 0 1 1-e 0+e 0+e],[0 1 1 1-e 1-e 0+e],c3);plot([0 1 1 0 0],[0 0 1 1 0]);disp('Weights');
  "IW{1,1}(5,:)'" : Constant  Value=[0.233135476636889882318115496673271991312503814697265625;-0.1685291948239770742912213563613477163016796112060546875;0.06303456679283829522386639609976555220782756805419921875;-0.194107861902167166956445498726679943501949310302734375;-0.03547526910071478745134498922197963111102581024169921875;-0.06369582581620177041958896779760834760963916778564453125;-0.11269664696295826622485236612192238681018352508544921875;0.2425664412841019024202893206165754236280918121337890625;0.10631632208512313553239181374010513536632061004638671875;-0.1096395902551357270926501996655133552849292755126953125;0.193165058837961034488017730836872942745685577392578125]
      mask Display: e = 0.06;c1 = [120 150 230]/255;c2 = ([120 150 230]+0)/383;c3 = ([120 150 230]+128)/383;patch([0 1 1 0],[0 0 1 1],c1);patch([0 1 1 1-e 1-e 0+e],[0 0 1 1-e 0+e 0+e],c2);patch([0 0 1 1-e 0+e 0+e],[0 1 1 1-e 1-e 0+e],c3);plot([0 1 1 0 0],[0 0 1 1 0]);disp('Weights');
  "IW{1,1}(6,:)'" : Constant  Value=[-0.01223626772421004989255255424041024525649845600128173828125;-0.16211453418429788708721162038273178040981292724609375;0.1141564710284695693953693762523471377789974212646484375;0.306047805263846950385442369224620051681995391845703125;0.0193626919215042457567133027396266697905957698822021484375;0.03708344957188268453673885005628108046948909759521484375;-0.049380269410432851839853896080967388115823268890380859375;0.20053257217748077234631409737630747258663177490234375;0.1091909120453779802328853065773728303611278533935546875;-0.06810787943101508090659734762084553949534893035888671875;0.267564548852841255222045901973615400493144989013671875]
      mask Display: e = 0.06;c1 = [120 150 230]/255;c2 = ([120 150 230]+0)/383;c3 = ([120 150 230]+128)/383;patch([0 1 1 0],[0 0 1 1],c1);patch([0 1 1 1-e 1-e 0+e],[0 0 1 1-e 0+e 0+e],c2);patch([0 0 1 1-e 0+e 0+e],[0 1 1 1-e 1-e 0+e],c3);plot([0 1 1 0 0],[0 0 1 1 0]);disp('Weights');
  "IW{1,1}(7,:)'" : Constant  Value=[0.176047610092069872766984417467028833925724029541015625;-0.0267132536874018222672333422451629303395748138427734375;0.0760793966877056637709841879768646322190761566162109375;0.12273330146821899433451363847780157811939716339111328125;-0.06294547059893300378075053913562442176043987274169921875;0.140876518826168861675540711075882427394390106201171875;0.1660035383030702416107260432909242808818817138671875;-0.06876639705224936449656780723671545274555683135986328125;-0.1664353175819342223196173335963976569473743438720703125;0.042721865086510955877852069306754856370389461517333984375;-0.16982874176570106339312360432813875377178192138671875]
      mask Display: e = 0.06;c1 = [120 150 230]/255;c2 = ([120 150 230]+0)/383;c3 = ([120 150 230]+128)/383;patch([0 1 1 0],[0 0 1 1],c1);patch([0 1 1 1-e 1-e 0+e],[0 0 1 1-e 0+e 0+e],c2);patch([0 0 1 1-e 0+e 0+e],[0 1 1 1-e 1-e 0+e],c3);plot([0 1 1 0 0],[0 0 1 1 0]);disp('Weights');
  "IW{1,1}(8,:)'" : Constant  Value=[-0.392582946572644309046751232017413713037967681884765625;-0.030979887039933741432751190814087749458849430084228515625;0.290967701752447072127694127630093134939670562744140625;0.1007823637899452340338513067763415165245532989501953125;0.08006739272746822566606539339773007668554782867431640625;0.023841213943834045629888152006969903595745563507080078125;-0.1088438690904235672807232049308368004858493804931640625;0.08370303420959290807701336234458722174167633056640625;-0.247325811799446848571193413590663112699985504150390625;0.0301913403509582213557482788246488780714571475982666015625;0.04142060306156343518768636613458511419594287872314453125]
      mask Display: e = 0.06;c1 = [120 150 230]/255;c2 = ([120 150 230]+0)/383;c3 = ([120 150 230]+128)/383;patch([0 1 1 0],[0 0 1 1],c1);patch([0 1 1 1-e 1-e 0+e],[0 0 1 1-e 0+e 0+e],c2);patch([0 0 1 1-e 0+e 0+e],[0 1 1 1-e 1-e 0+e],c3);plot([0 1 1 0 0],[0 0 1 1 0]);disp('Weights');
  "IW{1,1}(9,:)'" : Constant  Value=[0.253071923135122334169722080332576297223567962646484375;0.07268939423800346855131238044123165309429168701171875;0.0397677237833406194145169365583569742739200592041015625;-0.09207461253353839414348414038613555021584033966064453125;0.1260415550443266530233898947699344716966152191162109375;0.225409368345839411507114391497452743351459503173828125;0.1214058081603297811756903001878526993095874786376953125;-0.248321672667949300272738355488399975001811981201171875;-0.1597399561929817857208746545438771136105060577392578125;-0.075824478959162056046494626571075059473514556884765625;0.029458360811409324553356015030658454634249210357666015625]
      mask Display: e = 0.06;c1 = [120 150 230]/255;c2 = ([120 150 230]+0)/383;c3 = ([120 150 230]+128)/383;patch([0 1 1 0],[0 0 1 1],c1);patch([0 1 1 1-e 1-e 0+e],[0 0 1 1-e 0+e 0+e],c2);patch([0 0 1 1-e 0+e 0+e],[0 1 1 1-e 1-e 0+e],c3);plot([0 1 1 0 0],[0 0 1 1 0]);disp('Weights');
  Mux : Mux  Inputs=20
      mask Display: e = 0.06;c1 = [120 150 230]/255;c2 = ([120 150 230]+0)/383;c3 = ([120 150 230]+128)/383;patch([0 1 1 0],[0 0 1 1],c1);patch([0 1 1 1-e 1-e 0+e],[0 0 1 1-e 0+e 0+e],c2);patch([0 0 1 1-e 0+e 0+e],[0 1 1 1-e 1-e 0+e],c3);plot([0 1 1 0 0],[0 0 1 1 0]);disp('Mux');
  dotprod{1..20} (20 alike) : neural/Weight Functions/dotprod
  "iz{1,1}" : Outport
      mask Display: e = 0.06;c1 = [120 230 180]/255;c2 = ([120 230 180]+0)/(256+128);c3 = ([120 230 180]+128)/(256+128);patch([0 1 1 0],[0 0 1 1],c1);patch([0 1 1 1-e 1-e 0+e],[0 0 1 1-e 0+e 0+e],c2);patch([0 0 1 1-e 0+e 0+e],[0 1 1 1-e 1-e 0+e],c3);plot([0 1 1 0 0],[0 0 1 1 0]);
  wires:
  "IW{1,1}(1,:)'"/1 -> dotprod1/1
  "pd{1,1}"/1 -> dotprod1/2, dotprod2/2, dotprod3/2, dotprod4/2, dotprod5/2, dotprod6/2, dotprod7/2, dotprod8/2, dotprod9/2, dotprod10/2, dotprod11/2, dotprod12/2, dotprod13/2, dotprod14/2, dotprod15/2, dotprod16/2, dotprod17/2, dotprod18/2, dotprod19/2, dotprod20/2
  dotprod1/1 -> Mux/1
  "IW{1,1}(2,:)'"/1 -> dotprod2/1
  dotprod2/1 -> Mux/2
  "IW{1,1}(3,:)'"/1 -> dotprod3/1
  dotprod3/1 -> Mux/3
  "IW{1,1}(4,:)'"/1 -> dotprod4/1
  dotprod4/1 -> Mux/4
  "IW{1,1}(5,:)'"/1 -> dotprod5/1
  dotprod5/1 -> Mux/5
  "IW{1,1}(6,:)'"/1 -> dotprod6/1
  dotprod6/1 -> Mux/6
  "IW{1,1}(7,:)'"/1 -> dotprod7/1
  dotprod7/1 -> Mux/7
  "IW{1,1}(8,:)'"/1 -> dotprod8/1
  dotprod8/1 -> Mux/8
  "IW{1,1}(9,:)'"/1 -> dotprod9/1
  dotprod9/1 -> Mux/9
  "IW{1,1}(10,:)'"/1 -> dotprod10/1
  dotprod10/1 -> Mux/10
  "IW{1,1}(11,:)'"/1 -> dotprod11/1
  dotprod11/1 -> Mux/11
  "IW{1,1}(12,:)'"/1 -> dotprod12/1
  dotprod12/1 -> Mux/12
  "IW{1,1}(13,:)'"/1 -> dotprod13/1
  dotprod13/1 -> Mux/13
  "IW{1,1}(14,:)'"/1 -> dotprod14/1
  dotprod14/1 -> Mux/14
  "IW{1,1}(15,:)'"/1 -> dotprod15/1
  dotprod15/1 -> Mux/15
  "IW{1,1}(16,:)'"/1 -> dotprod16/1
  dotprod16/1 -> Mux/16
  "IW{1,1}(17,:)'"/1 -> dotprod17/1
  dotprod17/1 -> Mux/17
  "IW{1,1}(18,:)'"/1 -> dotprod18/1
  dotprod18/1 -> Mux/18
  "IW{1,1}(19,:)'"/1 -> dotprod19/1
  dotprod19/1 -> Mux/19
  "IW{1,1}(20,:)'"/1 -> dotprod20/1
  dotprod20/1 -> Mux/20
  Mux/1 -> "iz{1,1}"/1
